simulink model "conSys_2robots_1_vGPU_vR2014a"  (Simulink 8.3)
settings: Solver=FixedStepDiscrete  StartTime=0.0  StopTime=350  FixedStep=Ts  RelTol=1e-3
values from neighbouring files (symbols this model uses):
  ck = double(max(abs([par.q0_r1;par.q0_r2] - [par.q0r_r1;par.q0r_r2]))*20/7000 + 6)    [startUp_conSys_2robots_1_vGPU_vR2014a.m]    (also in startUp_conSys_2robots_1_vR2014a.m = max(abs([par.q0_r1;par.q0_r2] - [par.q0r_r1;par.q0r_r2]))*20; startUp_conSys_2robots_2_vR2014a.m = max(abs([par.q0_r1;par.q0_r2] - [par.q0r_r1;par.q0r_r2]))*20; startUp_conSys_2robots_3_vR2014a.m = max(abs([par.q0_r1;par.q0_r2] - [par.q0r_r1;par.q0r_r2]))*20; startUp_conSys_2robots_4_vR2014a.m = max(abs([par.q0_r1;par.q0_r2] - [par.q0r_r1;par.q0r_r2]))*20)
  d_0 = 2000    [startUp_conSys_2robots_1_vGPU_vR2014a.m]    (also in startUp_conSys_2robots_1_vR2014a.m = 200; startUp_conSys_2robots_2_vR2014a.m = 200; startUp_conSys_2robots_3_vR2014a.m; startUp_conSys_2robots_4_vR2014a.m = 200)
  do1r_0 = dthc_0 + dph1_0    (= 0.2)    [startUp_conSys_2robots_1_vGPU_vR2014a.m]    (also in startUp_conSys_2robots_1_vR2014a.m = 0; startUp_conSys_2robots_2_vR2014a.m = 0; startUp_conSys_2robots_3_vR2014a.m = 0; startUp_conSys_2robots_4_vR2014a.m = 0)
  do2r_0 = dthc_0 + dph2_0    (= -0.2)    [startUp_conSys_2robots_1_vGPU_vR2014a.m]    (also in startUp_conSys_2robots_1_vR2014a.m = 0; startUp_conSys_2robots_2_vR2014a.m = 0; startUp_conSys_2robots_3_vR2014a.m = 0; startUp_conSys_2robots_4_vR2014a.m = 0)
  dx1r_0 = dxc_0 + sin(thc_0)*dd_0 + d_0*cos(thc_0)*dthc_0    [startUp_conSys_2robots_1_vGPU_vR2014a.m]    (also in startUp_conSys_2robots_1_vR2014a.m; startUp_conSys_2robots_2_vR2014a.m; startUp_conSys_2robots_3_vR2014a.m; startUp_conSys_2robots_4_vR2014a.m)
  dx2r_0 = dxc_0 - sin(thc_0)*dd_0 - d_0*cos(thc_0)*dthc_0    [startUp_conSys_2robots_1_vGPU_vR2014a.m]    (also in startUp_conSys_2robots_1_vR2014a.m; startUp_conSys_2robots_2_vR2014a.m; startUp_conSys_2robots_3_vR2014a.m; startUp_conSys_2robots_4_vR2014a.m)
  dy1r_0 = dyc_0 + cos(thc_0)*dd_0 - d_0*sin(thc_0)*dthc_0    [startUp_conSys_2robots_1_vGPU_vR2014a.m]    (also in startUp_conSys_2robots_1_vR2014a.m; startUp_conSys_2robots_2_vR2014a.m; startUp_conSys_2robots_3_vR2014a.m; startUp_conSys_2robots_4_vR2014a.m)
  dy2r_0 = dyc_0 - cos(thc_0)*dd_0 + d_0*sin(thc_0)*dthc_0    [startUp_conSys_2robots_1_vGPU_vR2014a.m]    (also in startUp_conSys_2robots_1_vR2014a.m; startUp_conSys_2robots_2_vR2014a.m; startUp_conSys_2robots_3_vR2014a.m; startUp_conSys_2robots_4_vR2014a.m)
  o1r_0 = pi/2 - thc_0    (= 0)    [startUp_conSys_2robots_1_vGPU_vR2014a.m]    (also in startUp_conSys_2robots_1_vR2014a.m = pi/2 - thc_0; startUp_conSys_2robots_2_vR2014a.m = pi/2 - thc_0; startUp_conSys_2robots_3_vR2014a.m; startUp_conSys_2robots_4_vR2014a.m = th1_0)
  o2r_0 = pi/2 - thc_0    (= 0)    [startUp_conSys_2robots_1_vGPU_vR2014a.m]    (also in startUp_conSys_2robots_1_vR2014a.m = pi/2 - thc_0; startUp_conSys_2robots_2_vR2014a.m = pi/2 - thc_0; startUp_conSys_2robots_3_vR2014a.m; startUp_conSys_2robots_4_vR2014a.m = th2_0)
  thc_0 = pi/2    (= 1.57079632679)    [startUp_conSys_2robots_1_vGPU_vR2014a.m]    (also in startUp_conSys_2robots_1_vR2014a.m = atan2(1/25,1/12.5) + pi/2; startUp_conSys_2robots_2_vR2014a.m = atan2(1/25,1/12.5) + pi/2; startUp_conSys_2robots_3_vR2014a.m; startUp_conSys_2robots_4_vR2014a.m = atan2(1/25,1/12.5) + pi/2)
  Ts = 1/80    (= 0.0125)    [startUp_conSys_2robots_1_vGPU_vR2014a.m]    (also in startUp_conSys_2robots_1_vR2014a.m; startUp_conSys_2robots_2_vR2014a.m; startUp_conSys_2robots_3_vR2014a.m = 0.005; startUp_conSys_2robots_4_vR2014a.m = 0.005)
  x1_0 = 12000    [startUp_conSys_2robots_1_vGPU_vR2014a.m]    (also in startUp_conSys_2robots_1_vR2014a.m = 13178.9; startUp_conSys_2robots_2_vR2014a.m = 13178.9; startUp_conSys_2robots_3_vR2014a.m; startUp_conSys_2robots_4_vR2014a.m = 13178.9)
  x2_0 = 8000    [startUp_conSys_2robots_1_vGPU_vR2014a.m]    (also in startUp_conSys_2robots_1_vR2014a.m = 12821.1; startUp_conSys_2robots_2_vR2014a.m = 12821.1; startUp_conSys_2robots_3_vR2014a.m; startUp_conSys_2robots_4_vR2014a.m = 12821.1)
  xc_0 = 10000    [startUp_conSys_2robots_1_vGPU_vR2014a.m]    (also in startUp_conSys_2robots_1_vR2014a.m = 13000; startUp_conSys_2robots_2_vR2014a.m = 13000; startUp_conSys_2robots_3_vR2014a.m; startUp_conSys_2robots_4_vR2014a.m = 13000)
  y1_0 = 10000    [startUp_conSys_2robots_1_vGPU_vR2014a.m]    (also in startUp_conSys_2robots_1_vR2014a.m = 12910.6; startUp_conSys_2robots_2_vR2014a.m = 12910.6; startUp_conSys_2robots_3_vR2014a.m; startUp_conSys_2robots_4_vR2014a.m = 12910.6)
  y2_0 = 10000    [startUp_conSys_2robots_1_vGPU_vR2014a.m]    (also in startUp_conSys_2robots_1_vR2014a.m = 13089.4; startUp_conSys_2robots_2_vR2014a.m = 13089.4; startUp_conSys_2robots_3_vR2014a.m; startUp_conSys_2robots_4_vR2014a.m = 13089.4)
  yc_0 = 10000    [startUp_conSys_2robots_1_vGPU_vR2014a.m]    (also in startUp_conSys_2robots_1_vR2014a.m = 13000; startUp_conSys_2robots_2_vR2014a.m = 13000; startUp_conSys_2robots_3_vR2014a.m; startUp_conSys_2robots_4_vR2014a.m = 13000)
undefined symbols (not defined in the file or in its folder): absoluteAngle01_vR2014a, absoluteAngle02_vR2014a, DiscIntNeverNeededParam
undefined symbols (not defined in the file): ADAMS_cwd, ADAMS_exec, ADAMS_host, ADAMS_init, ADAMS_inputs, ADAMS_outputs, ADAMS_prefix, ADAMS_static, ADAMS_sysdir
libraries: simulink x18, cstblocks x7
(part 2 of 2)

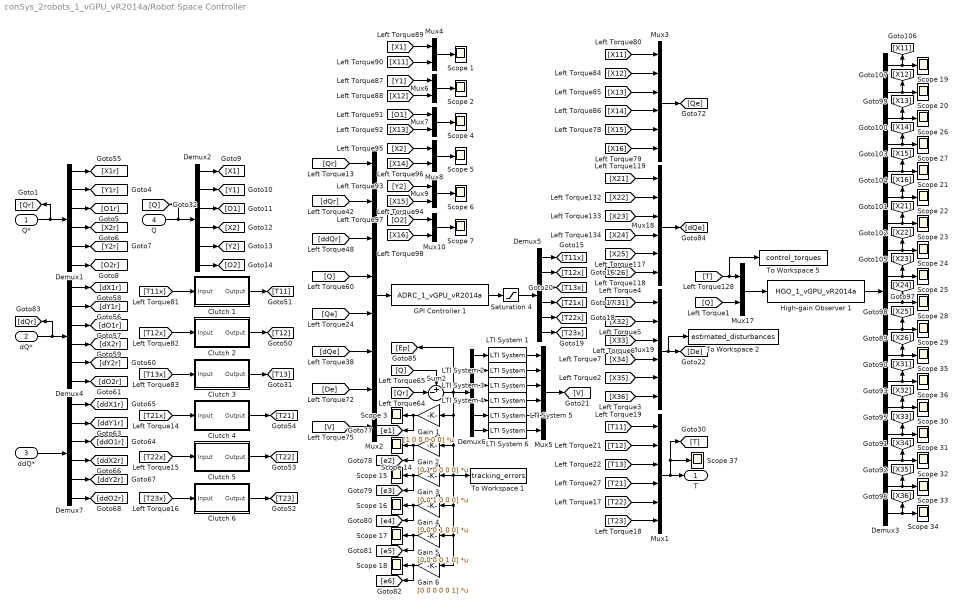
== system conSys_2robots_1_vGPU_vR2014a/Robot Space Controller ==
  Q* : Inport
  dQ* : Inport  Port=2
  ddQ* : Inport  Port=3
  Q : Inport  Port=4
  Clutch 1 : Subsystem
  Clutch 2 : Subsystem
  Clutch 3 : Subsystem
  Clutch 4 : Subsystem
  Clutch 5 : Subsystem
  Clutch 6 : Subsystem
  Demux{1..2,4..7} (6 alike) : Demux  Outputs=6
  Demux3 : Demux  Outputs=18
  GPI Controller 1 : S-Function  FunctionName=ADRC_1_vGPU_vR2014a  Parameters=par  EnableBusSupport=off
  Gain 1 : Gain  Gain=[1 0 0 0 0 0]  Multiplication=Matrix(K*u)
  Gain 2 : Gain  Gain=[0 1 0 0 0 0]  Multiplication=Matrix(K*u)
  Gain 3 : Gain  Gain=[0 0 1 0 0 0]  Multiplication=Matrix(K*u)
  Gain 4 : Gain  Gain=[0 0 0 1 0 0]  Multiplication=Matrix(K*u)
  Gain 5 : Gain  Gain=[0 0 0 0 1 0]  Multiplication=Matrix(K*u)
  Gain 6 : Gain  Gain=[0 0 0 0 0 1]  Multiplication=Matrix(K*u)
  High-gain Observer 1 : S-Function  FunctionName=HGO_1_vGPU_vR2014a  Parameters=par  EnableBusSupport=off
  LTI System {1..2,4..5} (4 alike) : cstblocks/LTI System  sys=par.Gz_1  IC=[]
  LTI System 3 : cstblocks/LTI System  sys=par.Gz_2  IC=[]
  LTI System 6 : cstblocks/LTI System  sys=par.Gz_2  IC=[]
  Mux{1,3,5,18..19} (5 alike) : Mux  Inputs=6
  Mux{4,6..10,17} (7 alike) : Mux  Inputs=2
  Mux2 : Mux  Inputs=8
  Saturation 4 : Saturate  UpperLimit=100  LowerLimit=-100
  Scope {1..7,14..37} (31 alike) : Scope
      Scope 1 settings: YMin=-2000  YMax=16000  SaveName=ScopeData37
      Scope 14 settings: YMin=-5000  YMax=1000  SaveName=ScopeData77
      Scope 15 settings: YMin=-1  YMax=10  SaveName=ScopeData78
      Scope 16 settings: YMin=-10000  YMax=1000  SaveName=ScopeData82
      Scope 17 settings: YMin=-1000  YMax=10000  SaveName=ScopeData83
      Scope 18 settings: YMin=-1  YMax=10  SaveName=ScopeData84
      Scope 19 settings: YMin=-2000  YMax=16000  SaveName=ScopeData86
      Scope 2 settings: YMin=-2000  YMax=16000  SaveName=ScopeData39
      Scope 20 settings: YMin=0  YMax=20000  SaveName=ScopeData87
      Scope 21 settings: YMin=0  YMax=5000  SaveName=ScopeData88
      Scope 22 settings: YMin=-100  YMax=200  SaveName=ScopeData90
      Scope 23 settings: YMin=-10  YMax=100  SaveName=ScopeData91
      Scope 24 settings: YMin=-50  YMax=50  SaveName=ScopeData92
      Scope 25 settings: YMin=-6  YMax=6  SaveName=ScopeData93
      Scope 26 settings: SaveName=ScopeData94
      Scope 27 settings: TimeRange=388  YMin=-1000  YMax=1000  SaveName=ScopeData95
      Scope 28 settings: YMin=0  YMax=10000  SaveName=ScopeData96
      Scope 29 settings: YMin=0  YMax=10000  SaveName=ScopeData97
      Scope 3 settings: YMin=-4000  YMax=1000  SaveName=ScopeData40
      Scope 30 settings: YMin=-300  YMax=300  SaveName=ScopeData98
      Scope 31 settings: YMin=-2  YMax=2  SaveName=ScopeData99
      Scope 32 settings: YMin=-300  YMax=300  SaveName=ScopeData100
      Scope 33 settings: YMin=-30  YMax=30  SaveName=ScopeData101
      Scope 34 settings: YMin=-4  SaveName=ScopeData102
      Scope 35 settings: SaveName=ScopeData103
      Scope 36 settings: YMin=-600  YMax=600  SaveName=ScopeData104
      Scope 37 settings: YMin=-100  YMax=100  SaveName=ScopeData119
      Scope 4 settings: YMin=-2  YMax=4  SaveName=ScopeData41
      Scope 5 settings: YMin=-2000  YMax=16000  SaveName=ScopeData43
      Scope 6 settings: YMin=-20  YMax=20  SaveName=ScopeData44
      Scope 7 settings: YMin=-20  YMax=20  SaveName=ScopeData45
  Sum2 : Sum  Inputs=+-|
  To Workspace 1 : ToWorkspace  VariableName=tracking_errors  SaveFormat=Structure With Time  SampleTime=-1
  To Workspace 2 : ToWorkspace  VariableName=estimated_disturbances  SaveFormat=Structure With Time  SampleTime=-1
  To Workspace 5 : ToWorkspace  VariableName=control_torques  SaveFormat=Structure With Time  SampleTime=-1
  T : Outport
  wires:
  Q/1 -> Demux2/1, [Q]
  Demux2/1 -> [X1]
  Demux2/2 -> [Y1]
  Demux2/3 -> [O1]
  Demux2/4 -> [X2]
  Demux2/5 -> [Y2]
  Demux2/6 -> [O2]
  Mux2/1 -> GPI Controller 1/1
  Demux5/1 -> [T11x]
  Demux5/2 -> [T12x]
  Demux5/3 -> [T13x]
  Saturation 4/1 -> Demux5/1
  Demux5/4 -> [T21x]
  Demux5/5 -> [T22x]
  Demux5/6 -> [T23x]
  [Qr] -> Sum2/2
  [Q] -> Sum2/1
  Demux6/1 -> LTI System 1/1
  Demux6/2 -> LTI System 2/1
  Demux6/3 -> LTI System 3/1
  [T11x] -> Clutch 1/1(Input)
  Clutch 1/1(Output) -> [T11]
  [T12x] -> Clutch 2/1(Input)
  Clutch 2/1(Output) -> [T12]
  [T13x] -> Clutch 3/1(Input)
  Clutch 3/1(Output) -> [T13]
  [T21x] -> Clutch 4/1(Input)
  Clutch 4/1(Output) -> [T21]
  [T22x] -> Clutch 5/1(Input)
  Clutch 5/1(Output) -> [T22]
  [T23x] -> Clutch 6/1(Input)
  Clutch 6/1(Output) -> [T23]
  [T11] -> Mux1/1
  [T23] -> Mux1/6
  [T21] -> Mux1/4
  [T22] -> Mux1/5
  [T12] -> Mux1/2
  [T13] -> Mux1/3
  Mux1/1 -> [T], Scope 37/1, T/1
  Q*/1 -> [Qr], Demux1/1
  Demux1/1 -> [X1r]
  Demux1/2 -> [Y1r]
  Demux1/3 -> [O1r]
  Demux1/4 -> [X2r]
  Demux1/5 -> [Y2r]
  Demux1/6 -> [O2r]
  dQ*/1 -> [dQr], Demux4/1
  Demux4/1 -> [dX1r]
  Demux4/2 -> [dY1r]
  Demux4/3 -> [dO1r]
  Demux4/4 -> [dX2r]
  Demux4/5 -> [dY2r]
  Demux4/6 -> [dO2r]
  Demux7/1 -> [ddX1r]
  Demux7/2 -> [ddY1r]
  Demux7/3 -> [ddO1r]
  Demux7/4 -> [ddX2r]
  Demux7/5 -> [ddY2r]
  Demux7/6 -> [ddO2r]
  ddQ*/1 -> Demux7/1
  Demux6/4 -> LTI System 4/1
  Demux6/5 -> LTI System 5/1
  Demux6/6 -> LTI System 6/1
  [X11] -> Mux3/1
  [X16] -> Mux3/6
  [X14] -> Mux3/4
  [X15] -> Mux3/5
  [X12] -> Mux3/2
  [X13] -> Mux3/3
  Mux3/1 -> [Qe]
  [X11] -> Mux4/2
  [X1] -> Mux4/1
  Mux4/1 -> Scope 1/1
  [X12] -> Mux6/2
  [Y1] -> Mux6/1
  Mux6/1 -> Scope 2/1
  [X13] -> Mux7/2
  [O1] -> Mux7/1
  Mux7/1 -> Scope 4/1
  [X14] -> Mux8/2
  [X2] -> Mux8/1
  Mux8/1 -> Scope 5/1
  [X15] -> Mux9/2
  [Y2] -> Mux9/1
  Mux9/1 -> Scope 6/1
  [X16] -> Mux10/2
  [O2] -> Mux10/1
  Mux10/1 -> Scope 7/1
  LTI System 1/1 -> Mux5/1
  LTI System 2/1 -> Mux5/2
  LTI System 3/1 -> Mux5/3
  LTI System 4/1 -> Mux5/4
  LTI System 5/1 -> Mux5/5
  LTI System 6/1 -> Mux5/6
  Gain 1/1 -> [e1], Scope 3/1
  Gain 2/1 -> [e2], Scope 14/1
  Gain 3/1 -> [e3], Scope 15/1
  Gain 4/1 -> [e4], Scope 16/1
  Gain 5/1 -> [e5], Scope 17/1
  Sum2/1 -> [Ep], Demux6/1, To Workspace 1/1, Gain 6/1, Gain 5/1, Gain 4/1, Gain 3/1, Gain 2/1, Gain 1/1
  Gain 6/1 -> [e6], Scope 18/1
  Mux17/1 -> High-gain Observer 1/1
  Demux3/9 -> Scope 25/1, [X23]
  Demux3/7 -> [X21], Scope 23/1
  Demux3/8 -> [X22], Scope 24/1
  Demux3/5 -> [X15], Scope 21/1
  Demux3/6 -> [X16], Scope 22/1
  High-gain Observer 1/1 -> Demux3/1
  Demux3/3 -> Scope 26/1, [X13]
  Demux3/4 -> Scope 27/1, [X14]
  Demux3/1 -> Scope 19/1, [X11]
  Demux3/2 -> Scope 20/1, [X12]
  Demux3/17 -> Scope 33/1, [X35]
  Demux3/13 -> [X31], Scope 36/1
  Demux3/12 -> [X26], Scope 35/1
  Demux3/18 -> [X36], Scope 34/1
  Demux3/15 -> Scope 31/1, [X33]
  Demux3/10 -> [X24], Scope 28/1
  Demux3/11 -> [X25], Scope 29/1
  Demux3/16 -> Scope 32/1, [X34]
  Demux3/14 -> Scope 30/1, [X32]
  [X21] -> Mux18/1
  [X26] -> Mux18/6
  [X24] -> Mux18/4
  [X25] -> Mux18/5
  [X22] -> Mux18/2
  [X23] -> Mux18/3
  Mux18/1 -> [dQe]
  [Q] -> Mux17/2
  Mux5/1 -> [V]
  [Qr] -> Mux2/1
  [Qe] -> Mux2/5
  [dQe] -> Mux2/6
  [dQr] -> Mux2/2
  [ddQr] -> Mux2/3
  [Q] -> Mux2/4
  [De] -> Mux2/7
  [V] -> Mux2/8
  [X31] -> Mux19/1
  [X36] -> Mux19/6
  [X34] -> Mux19/4
  [X35] -> Mux19/5
  [X32] -> Mux19/2
  [X33] -> Mux19/3
  Mux19/1 -> To Workspace 2/1, [De]
  GPI Controller 1/1 -> Saturation 4/1
  [T] -> To Workspace 5/1, Mux17/1

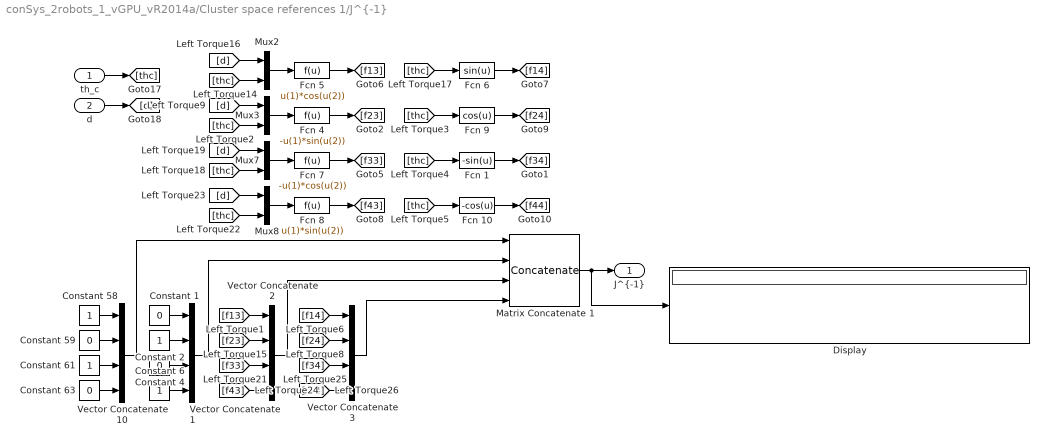
== system conSys_2robots_1_vGPU_vR2014a/Cluster space references 1/J^{-1} ==
  th_c : Inport
  d : Inport  Port=2
  Constant {1,4,59,63} (4 alike) : Constant  Value=0
  Constant {2,6,58,61} (4 alike) : Constant
  Display : Display
  Fcn 1 : Fcn  Expr=-sin(u)
  Fcn 10 : Fcn  Expr=-cos(u)
  Fcn 4 : Fcn  Expr=-u(1)*sin(u(2))
  Fcn 5 : Fcn  Expr=u(1)*cos(u(2))
  Fcn 6 : Fcn  Expr=sin(u)
  Fcn 7 : Fcn  Expr=-u(1)*cos(u(2))
  Fcn 8 : Fcn  Expr=u(1)*sin(u(2))
  Fcn 9 : Fcn  Expr=cos(u)
  Matrix Concatenate 1 : Concatenate  NumInputs=4  Mode=Multidimensional array  ConcatenateDimension=2
  Mux{2..3,7..8} (4 alike) : Mux  Inputs=2
  Vector Concatenate {1..3,10} (4 alike) : Concatenate  NumInputs=4
  "J^{-1}" : Outport
  wires:
  d/1 -> [d]
  th_c/1 -> [thc]
  Matrix Concatenate 1/1 -> "J^{-1}"/1, Display/1
  Vector Concatenate 10/1 -> Matrix Concatenate 1/1
  Vector Concatenate 1/1 -> Matrix Concatenate 1/2
  Vector Concatenate 2/1 -> Matrix Concatenate 1/3
  Constant 58/1 -> Vector Concatenate 10/1
  Constant 59/1 -> Vector Concatenate 10/2
  Constant 61/1 -> Vector Concatenate 10/3
  Constant 63/1 -> Vector Concatenate 10/4
  Constant 1/1 -> Vector Concatenate 1/1
  Constant 2/1 -> Vector Concatenate 1/2
  Constant 4/1 -> Vector Concatenate 1/3
  Constant 6/1 -> Vector Concatenate 1/4
  Vector Concatenate 3/1 -> Matrix Concatenate 1/4
  [d] -> Mux2/1
  [thc] -> Mux2/2
  Mux2/1 -> Fcn 5/1
  Fcn 5/1 -> [f13]
  Fcn 6/1 -> [f14]
  [thc] -> Fcn 6/1
  [f13] -> Vector Concatenate 2/1
  [d] -> Mux3/1
  [thc] -> Mux3/2
  Mux3/1 -> Fcn 4/1
  Fcn 4/1 -> [f23]
  [f23] -> Vector Concatenate 2/2
  [d] -> Mux7/1
  [thc] -> Mux7/2
  Mux7/1 -> Fcn 7/1
  Fcn 7/1 -> [f33]
  [f33] -> Vector Concatenate 2/3
  [d] -> Mux8/1
  [thc] -> Mux8/2
  Mux8/1 -> Fcn 8/1
  Fcn 8/1 -> [f43]
  [f43] -> Vector Concatenate 2/4
  Fcn 9/1 -> [f24]
  [thc] -> Fcn 9/1
  Fcn 1/1 -> [f34]
  [thc] -> Fcn 1/1
  Fcn 10/1 -> [f44]
  [thc] -> Fcn 10/1
  [f14] -> Vector Concatenate 3/1
  [f24] -> Vector Concatenate 3/2
  [f34] -> Vector Concatenate 3/3
  [f44] -> Vector Concatenate 3/4

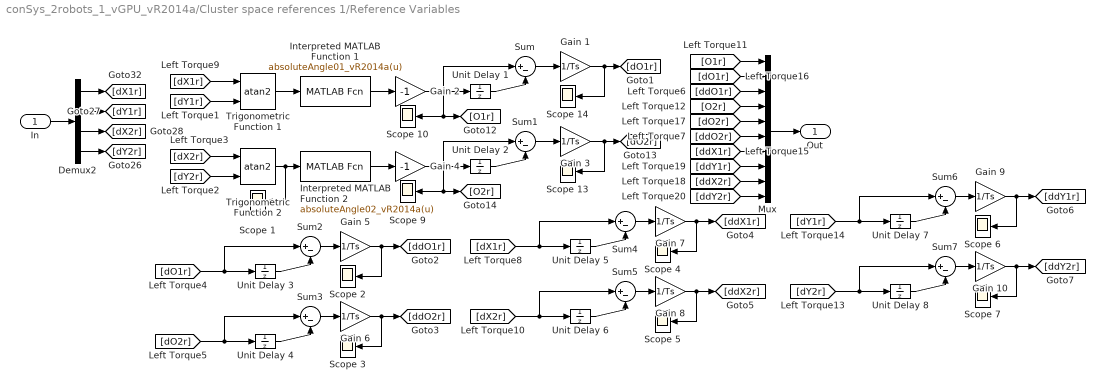
== system conSys_2robots_1_vGPU_vR2014a/Cluster space references 1/Reference Variables ==
  In : Inport  PortDimensions=4
  Demux2 : Demux
  Gain {1,3,5..10} (8 alike) : Gain  Gain=1/Ts
  Gain 2 : Gain  Gain=-1
  Gain 4 : Gain  Gain=-1
  Interpreted MATLAB Function 1 : MATLABFcn  MATLABFcn=absoluteAngle01_vR2014a(u)
  Interpreted MATLAB Function 2 : MATLABFcn  MATLABFcn=absoluteAngle02_vR2014a(u)
  Mux : Mux  Inputs=10
  Scope {1..7,9..10,13..14} (11 alike) : Scope
      Scope 1 settings: YMin=0  YMax=10  SaveName=ScopeData61
      Scope 10 settings: TimeRange=500  YMin=-15  YMax=15  SaveName=ScopeData68
      Scope 13 settings: YMin=-0.45  YMax=0.47  SaveName=ScopeData71
      Scope 14 settings: YMin=-0.45  YMax=0.47  SaveName=ScopeData72
      Scope 2 settings: YMin=-0.02  YMax=0.02  SaveName=ScopeData26
      Scope 3 settings: YMin=-0.45  YMax=0.47  SaveName=ScopeData27
      Scope 4 settings: YMin=-0.02  YMax=0.02  SaveName=ScopeData55
      Scope 5 settings: YMin=-0.45  YMax=0.47  SaveName=ScopeData56
      Scope 6 settings: YMin=-0.02  YMax=0.02  SaveName=ScopeData57
      Scope 7 settings: YMin=-0.45  YMax=0.47  SaveName=ScopeData58
      Scope 9 settings: YMin=-10  YMax=10  SaveName=ScopeData67
  Sum{,1..7} (8 alike) : Sum  Inputs=|+-
  Trigonometric Function 1 : Trigonometry  Operator=atan2
  Trigonometric Function 2 : Trigonometry  Operator=atan2
  Unit Delay 1 : UnitDelay  InitialCondition=o1r_0  SampleTime=-1
  Unit Delay 2 : UnitDelay  InitialCondition=o2r_0  SampleTime=-1
  Unit Delay 3 : UnitDelay  InitialCondition=do1r_0  SampleTime=-1
  Unit Delay 4 : UnitDelay  InitialCondition=do2r_0  SampleTime=-1
  Unit Delay 5 : UnitDelay  InitialCondition=dx1r_0  SampleTime=-1
  Unit Delay 6 : UnitDelay  InitialCondition=dx2r_0  SampleTime=-1
  Unit Delay 7 : UnitDelay  InitialCondition=dy1r_0  SampleTime=-1
  Unit Delay 8 : UnitDelay  InitialCondition=dy2r_0  SampleTime=-1
  Out : Outport  PortDimensions=10
  wires:
  In/1 -> Demux2/1
  Demux2/1 -> [dX1r]
  Demux2/2 -> [dY1r]
  Demux2/3 -> [dX2r]
  Demux2/4 -> [dY2r]
  [dX1r] -> Trigonometric Function 1/1
  [dY1r] -> Trigonometric Function 1/2
  Interpreted MATLAB Function 1/1 -> Gain 2/1
  Unit Delay 1/1 -> Sum/2
  Sum/1 -> Gain 1/1
  Gain 1/1 -> Scope 14/1, [dO1r]
  Trigonometric Function 1/1 -> Interpreted MATLAB Function 1/1
  Gain 2/1 -> Scope 10/1, [O1r], Sum/1, Unit Delay 1/1
  [dX2r] -> Trigonometric Function 2/1
  [dY2r] -> Trigonometric Function 2/2
  Interpreted MATLAB Function 2/1 -> Gain 4/1
  Unit Delay 2/1 -> Sum1/2
  Sum1/1 -> Gain 3/1
  Gain 3/1 -> Scope 13/1, [dO2r]
  Trigonometric Function 2/1 -> Scope 1/1, Interpreted MATLAB Function 2/1
  Gain 4/1 -> Unit Delay 2/1, Sum1/1, Scope 9/1, [O2r]
  Mux/1 -> Out/1
  Unit Delay 3/1 -> Sum2/2
  Sum2/1 -> Gain 5/1
  Gain 5/1 -> Scope 2/1, [ddO1r]
  Unit Delay 4/1 -> Sum3/2
  Sum3/1 -> Gain 6/1
  Gain 6/1 -> [ddO2r], Scope 3/1
  [O1r] -> Mux/1
  [dO1r] -> Mux/2
  [dO2r] -> Mux/5
  [O2r] -> Mux/4
  [ddO1r] -> Mux/3
  [ddO2r] -> Mux/6
  [dO1r] -> Sum2/1, Unit Delay 3/1
  [dO2r] -> Unit Delay 4/1, Sum3/1
  Unit Delay 5/1 -> Sum4/2
  Sum4/1 -> Gain 7/1
  Gain 7/1 -> [ddX1r], Scope 4/1
  Unit Delay 6/1 -> Sum5/2
  Sum5/1 -> Gain 8/1
  Gain 8/1 -> Scope 5/1, [ddX2r]
  [dX1r] -> Unit Delay 5/1, Sum4/1
  [dX2r] -> Sum5/1, Unit Delay 6/1
  Unit Delay 7/1 -> Sum6/2
  Sum6/1 -> Gain 9/1
  Gain 9/1 -> Scope 6/1, [ddY1r]
  Unit Delay 8/1 -> Sum7/2
  Sum7/1 -> Gain 10/1
  Gain 10/1 -> [ddY2r], Scope 7/1
  [dY1r] -> Sum6/1, Unit Delay 7/1
  [dY2r] -> Unit Delay 8/1, Sum7/1
  [ddX1r] -> Mux/7
  [ddY2r] -> Mux/10
  [ddY1r] -> Mux/8
  [ddX2r] -> Mux/9

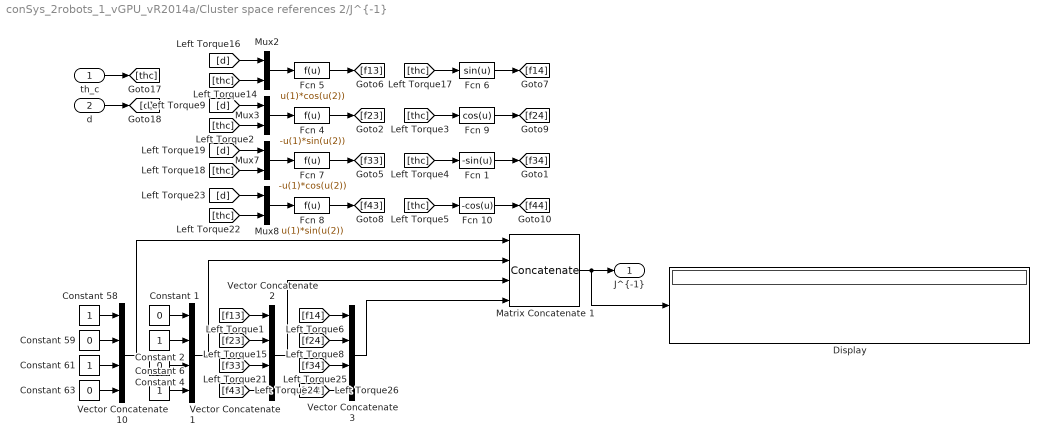
== system conSys_2robots_1_vGPU_vR2014a/Cluster space references 2/J^{-1} ==
  th_c : Inport
  d : Inport  Port=2
  Constant {1,4,59,63} (4 alike) : Constant  Value=0
  Constant {2,6,58,61} (4 alike) : Constant
  Display : Display
  Fcn 1 : Fcn  Expr=-sin(u)
  Fcn 10 : Fcn  Expr=-cos(u)
  Fcn 4 : Fcn  Expr=-u(1)*sin(u(2))
  Fcn 5 : Fcn  Expr=u(1)*cos(u(2))
  Fcn 6 : Fcn  Expr=sin(u)
  Fcn 7 : Fcn  Expr=-u(1)*cos(u(2))
  Fcn 8 : Fcn  Expr=u(1)*sin(u(2))
  Fcn 9 : Fcn  Expr=cos(u)
  Matrix Concatenate 1 : Concatenate  NumInputs=4  Mode=Multidimensional array  ConcatenateDimension=2
  Mux{2..3,7..8} (4 alike) : Mux  Inputs=2
  Vector Concatenate {1..3,10} (4 alike) : Concatenate  NumInputs=4
  "J^{-1}" : Outport
  wires:
  d/1 -> [d]
  th_c/1 -> [thc]
  Matrix Concatenate 1/1 -> "J^{-1}"/1, Display/1
  Vector Concatenate 10/1 -> Matrix Concatenate 1/1
  Vector Concatenate 1/1 -> Matrix Concatenate 1/2
  Vector Concatenate 2/1 -> Matrix Concatenate 1/3
  Constant 58/1 -> Vector Concatenate 10/1
  Constant 59/1 -> Vector Concatenate 10/2
  Constant 61/1 -> Vector Concatenate 10/3
  Constant 63/1 -> Vector Concatenate 10/4
  Constant 1/1 -> Vector Concatenate 1/1
  Constant 2/1 -> Vector Concatenate 1/2
  Constant 4/1 -> Vector Concatenate 1/3
  Constant 6/1 -> Vector Concatenate 1/4
  Vector Concatenate 3/1 -> Matrix Concatenate 1/4
  [d] -> Mux2/1
  [thc] -> Mux2/2
  Mux2/1 -> Fcn 5/1
  Fcn 5/1 -> [f13]
  Fcn 6/1 -> [f14]
  [thc] -> Fcn 6/1
  [f13] -> Vector Concatenate 2/1
  [d] -> Mux3/1
  [thc] -> Mux3/2
  Mux3/1 -> Fcn 4/1
  Fcn 4/1 -> [f23]
  [f23] -> Vector Concatenate 2/2
  [d] -> Mux7/1
  [thc] -> Mux7/2
  Mux7/1 -> Fcn 7/1
  Fcn 7/1 -> [f33]
  [f33] -> Vector Concatenate 2/3
  [d] -> Mux8/1
  [thc] -> Mux8/2
  Mux8/1 -> Fcn 8/1
  Fcn 8/1 -> [f43]
  [f43] -> Vector Concatenate 2/4
  Fcn 9/1 -> [f24]
  [thc] -> Fcn 9/1
  Fcn 1/1 -> [f34]
  [thc] -> Fcn 1/1
  Fcn 10/1 -> [f44]
  [thc] -> Fcn 10/1
  [f14] -> Vector Concatenate 3/1
  [f24] -> Vector Concatenate 3/2
  [f34] -> Vector Concatenate 3/3
  [f44] -> Vector Concatenate 3/4

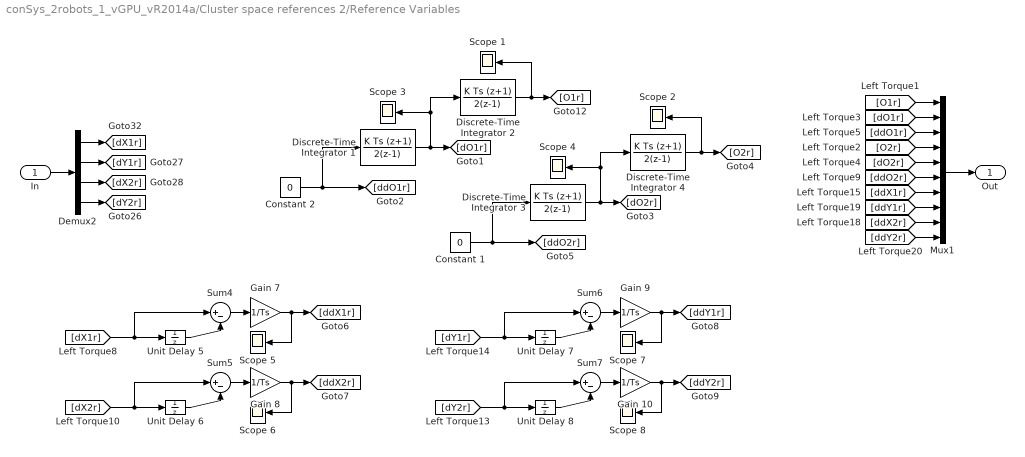
== system conSys_2robots_1_vGPU_vR2014a/Cluster space references 2/Reference Variables ==
  In : Inport  PortDimensions=4
  Constant 1 : Constant  Value=0
  Constant 2 : Constant  Value=0
  Demux2 : Demux
  Discrete-Time Integrator 1 : DiscreteIntegrator  IntegratorMethod=Integration: Trapezoidal  InitialCondition=do1r_0  SampleTime=Ts  ICPrevOutput=DiscIntNeverNeededParam  ICPrevScaledInput=DiscIntNeverNeededParam
  Discrete-Time Integrator 2 : DiscreteIntegrator  IntegratorMethod=Integration: Trapezoidal  InitialCondition=o1r_0  SampleTime=Ts  ICPrevOutput=DiscIntNeverNeededParam  ICPrevScaledInput=DiscIntNeverNeededParam
  Discrete-Time Integrator 3 : DiscreteIntegrator  IntegratorMethod=Integration: Trapezoidal  InitialCondition=do2r_0  SampleTime=Ts  ICPrevOutput=DiscIntNeverNeededParam  ICPrevScaledInput=DiscIntNeverNeededParam
  Discrete-Time Integrator 4 : DiscreteIntegrator  IntegratorMethod=Integration: Trapezoidal  InitialCondition=o2r_0  SampleTime=Ts  ICPrevOutput=DiscIntNeverNeededParam  ICPrevScaledInput=DiscIntNeverNeededParam
  Gain {7..10} (4 alike) : Gain  Gain=1/Ts
  Mux1 : Mux  Inputs=10
  Scope {1..8} (8 alike) : Scope
      Scope 1 settings: YMin=-0.45  YMax=0.47  SaveName=ScopeData18
      Scope 2 settings: YMin=-10  YMax=10  SaveName=ScopeData19
      Scope 3 settings: YMin=-0.45  YMax=0.47  SaveName=ScopeData27
      Scope 4 settings: YMin=-0.45  YMax=0.47  SaveName=ScopeData20
      Scope 5 settings: YMin=-0.02  YMax=0.02  SaveName=ScopeData21
      Scope 6 settings: YMin=-0.45  YMax=0.47  SaveName=ScopeData22
      Scope 7 settings: YMin=-0.02  YMax=0.02  SaveName=ScopeData23
      Scope 8 settings: YMin=-0.45  YMax=0.47  SaveName=ScopeData24
  Sum{4..7} (4 alike) : Sum  Inputs=|+-
  Unit Delay 5 : UnitDelay  InitialCondition=dx1r_0  SampleTime=-1
  Unit Delay 6 : UnitDelay  InitialCondition=dx2r_0  SampleTime=-1
  Unit Delay 7 : UnitDelay  InitialCondition=dy1r_0  SampleTime=-1
  Unit Delay 8 : UnitDelay  InitialCondition=dy2r_0  SampleTime=-1
  Out : Outport  PortDimensions=10
  wires:
  Constant 2/1 -> Discrete-Time Integrator 1/1, [ddO1r]
  Discrete-Time Integrator 1/1 -> Discrete-Time Integrator 2/1, Scope 3/1, [dO1r]
  Discrete-Time Integrator 2/1 -> Scope 1/1, [O1r]
  Constant 1/1 -> [ddO2r], Discrete-Time Integrator 3/1
  Discrete-Time Integrator 3/1 -> [dO2r], Scope 4/1, Discrete-Time Integrator 4/1
  Discrete-Time Integrator 4/1 -> [O2r], Scope 2/1
  In/1 -> Demux2/1
  Demux2/1 -> [dX1r]
  Demux2/2 -> [dY1r]
  Demux2/3 -> [dX2r]
  Demux2/4 -> [dY2r]
  Unit Delay 5/1 -> Sum4/2
  Sum4/1 -> Gain 7/1
  Gain 7/1 -> [ddX1r], Scope 5/1
  Unit Delay 6/1 -> Sum5/2
  Sum5/1 -> Gain 8/1
  Gain 8/1 -> Scope 6/1, [ddX2r]
  [dX1r] -> Unit Delay 5/1, Sum4/1
  [dX2r] -> Sum5/1, Unit Delay 6/1
  Unit Delay 7/1 -> Sum6/2
  Sum6/1 -> Gain 9/1
  Gain 9/1 -> Scope 7/1, [ddY1r]
  Unit Delay 8/1 -> Sum7/2
  Sum7/1 -> Gain 10/1
  Gain 10/1 -> [ddY2r], Scope 8/1
  [dY1r] -> Sum6/1, Unit Delay 7/1
  [dY2r] -> Unit Delay 8/1, Sum7/1
  Mux1/1 -> Out/1
  [O1r] -> Mux1/1
  [dO1r] -> Mux1/2
  [dO2r] -> Mux1/5
  [O2r] -> Mux1/4
  [ddO1r] -> Mux1/3
  [ddO2r] -> Mux1/6
  [ddX1r] -> Mux1/7
  [ddY2r] -> Mux1/10
  [ddY1r] -> Mux1/8
  [ddX2r] -> Mux1/9

== system conSys_2robots_1_vGPU_vR2014a/Omni Two-Robot ADAMS Model v2015/ADAMS Plant ==
  ADAMS inputs : Inport
  S-Function : S-Function  StopFcn=clear mex  FunctionName=adams_plant  Parameters=exevie,exesol,stat,outfil,nampre,o_rate,nam_in,namout,dft,modsim,modani,dt_out,inicmd,exetyp,comtyp,ada_host, workdir,pin_interp_order,pout_extrap_order,pin_extrap_order,pout_interp_order,simulink_lead_cosim  EnableBusSupport=off
  ADAMS outputs : Outport  InitialOutput=0
  wires:
  S-Function/1 -> ADAMS outputs/1
  ADAMS inputs/1 -> S-Function/1

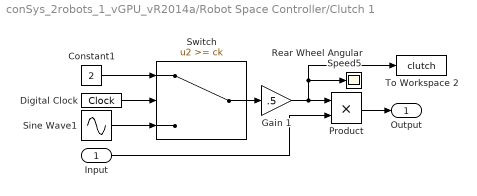
== system conSys_2robots_1_vGPU_vR2014a/Robot Space Controller/Clutch 1 ==
  Input : Inport
  Constant1 : Constant  Value=2
  Digital Clock : DigitalClock  SampleTime=Ts
  Gain 1 : Gain  Gain=.5
  Product : Product
  Rear Wheel Angular Speed5 : Scope
      settings: YMin=0  YMax=2  SaveName=ScopeData5
  Sine Wave1 : Sin  Bias=1  Frequency=(pi/ck)  Phase=-pi/2  SampleTime=Ts
  Switch : Switch  Threshold=ck
  To Workspace 2 : ToWorkspace  VariableName=clutch  SaveFormat=Structure With Time  SampleTime=-1
  Output : Outport
  wires:
  Constant1/1 -> Switch/1
  Digital Clock/1 -> Switch/2
  Switch/1 -> Gain 1/1
  Input/1 -> Product/2
  Product/1 -> Output/1
  Sine Wave1/1 -> Switch/3
  Gain 1/1 -> Rear Wheel Angular Speed5/1, To Workspace 2/1, Product/1

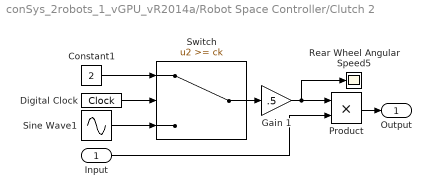
== system conSys_2robots_1_vGPU_vR2014a/Robot Space Controller/Clutch 2 ==
  Input : Inport
  Constant1 : Constant  Value=2
  Digital Clock : DigitalClock  SampleTime=Ts
  Gain 1 : Gain  Gain=.5
  Product : Product
  Rear Wheel Angular Speed5 : Scope
      settings: YMin=0  YMax=2  SaveName=ScopeData5
  Sine Wave1 : Sin  Bias=1  Frequency=(pi/ck)  Phase=-pi/2  SampleTime=Ts
  Switch : Switch  Threshold=ck
  Output : Outport
  wires:
  Gain 1/1 -> Product/1, Rear Wheel Angular Speed5/1
  Sine Wave1/1 -> Switch/3
  Product/1 -> Output/1
  Input/1 -> Product/2
  Switch/1 -> Gain 1/1
  Digital Clock/1 -> Switch/2
  Constant1/1 -> Switch/1

== system conSys_2robots_1_vGPU_vR2014a/Robot Space Controller/Clutch 3 ==
  Input : Inport
  Constant1 : Constant  Value=2
  Digital Clock : DigitalClock  SampleTime=Ts
  Gain 1 : Gain  Gain=.5
  Product : Product
  Rear Wheel Angular Speed5 : Scope
      settings: YMin=0  YMax=2  SaveName=ScopeData5
  Sine Wave1 : Sin  Bias=1  Frequency=(pi/ck)  Phase=-pi/2  SampleTime=Ts
  Switch : Switch  Threshold=ck
  Output : Outport
  wires:
  Constant1/1 -> Switch/1
  Digital Clock/1 -> Switch/2
  Switch/1 -> Gain 1/1
  Input/1 -> Product/2
  Product/1 -> Output/1
  Sine Wave1/1 -> Switch/3
  Gain 1/1 -> Rear Wheel Angular Speed5/1, Product/1

== system conSys_2robots_1_vGPU_vR2014a/Robot Space Controller/Clutch 4 ==
  Input : Inport
  Constant1 : Constant  Value=2
  Digital Clock : DigitalClock  SampleTime=Ts
  Gain 1 : Gain  Gain=.5
  Product : Product
  Rear Wheel Angular Speed5 : Scope
      settings: YMin=0  YMax=2  SaveName=ScopeData5
  Sine Wave1 : Sin  Bias=1  Frequency=(pi/ck)  Phase=-pi/2  SampleTime=Ts
  Switch : Switch  Threshold=ck
  Output : Outport
  wires:
  Gain 1/1 -> Product/1, Rear Wheel Angular Speed5/1
  Sine Wave1/1 -> Switch/3
  Product/1 -> Output/1
  Input/1 -> Product/2
  Switch/1 -> Gain 1/1
  Digital Clock/1 -> Switch/2
  Constant1/1 -> Switch/1

== system conSys_2robots_1_vGPU_vR2014a/Robot Space Controller/Clutch 5 ==
  Input : Inport
  Constant1 : Constant  Value=2
  Digital Clock : DigitalClock  SampleTime=Ts
  Gain 1 : Gain  Gain=.5
  Product : Product
  Rear Wheel Angular Speed5 : Scope
      settings: YMin=0  YMax=2  SaveName=ScopeData5
  Sine Wave1 : Sin  Bias=1  Frequency=(pi/ck)  Phase=-pi/2  SampleTime=Ts
  Switch : Switch  Threshold=ck
  Output : Outport
  wires:
  Constant1/1 -> Switch/1
  Digital Clock/1 -> Switch/2
  Switch/1 -> Gain 1/1
  Input/1 -> Product/2
  Product/1 -> Output/1
  Sine Wave1/1 -> Switch/3
  Gain 1/1 -> Rear Wheel Angular Speed5/1, Product/1

== system conSys_2robots_1_vGPU_vR2014a/Robot Space Controller/Clutch 6 ==
  Input : Inport
  Constant1 : Constant  Value=2
  Digital Clock : DigitalClock  SampleTime=Ts
  Gain 1 : Gain  Gain=.5
  Product : Product
  Rear Wheel Angular Speed5 : Scope
      settings: YMin=0  YMax=2  SaveName=ScopeData5
  Sine Wave1 : Sin  Bias=1  Frequency=(pi/ck)  Phase=-pi/2  SampleTime=Ts
  Switch : Switch  Threshold=ck
  Output : Outport
  wires:
  Gain 1/1 -> Product/1, Rear Wheel Angular Speed5/1
  Sine Wave1/1 -> Switch/3
  Product/1 -> Output/1
  Input/1 -> Product/2
  Switch/1 -> Gain 1/1
  Digital Clock/1 -> Switch/2
  Constant1/1 -> Switch/1
